simulink model "Modelo_nolineal_2GDL_2021"  (R2021b)
settings: Solver=VariableStepAuto  StartTime=0.0  StopTime=5  FixedStep=T  RelTol=1e-3
values from neighbouring files (symbols this model uses):
  g = 9.81    [initializationControl.m]
  Iyy = pod.mass.inertia(2,2)    [initializationControl.m]
  m = pod.mass.mass    [initializationControl.m]
  theta0 = 0    [initializationControl.m]
  x_lev = pod.geometry.x_LEV    [initializationControl.m]
  z_ini = z_0 + z_lev    [initializationControl.m]
  z_lev = pod.geometry.z_LEV    [initializationControl.m]
undefined symbols (not defined in the file or in its folder): k1, k2, k3, k4, p1, p2
settings Model: Creator=EDMAOR  LastModifiedBy=emate
settings SolverCC: AlgebraicLoopSolver=TrustRegion
settings DebuggingCC: SFMachineParentedDataDiag=warning
settings SFSimCC: CustomCodeUndefinedFunction=UseInterfaceOnly

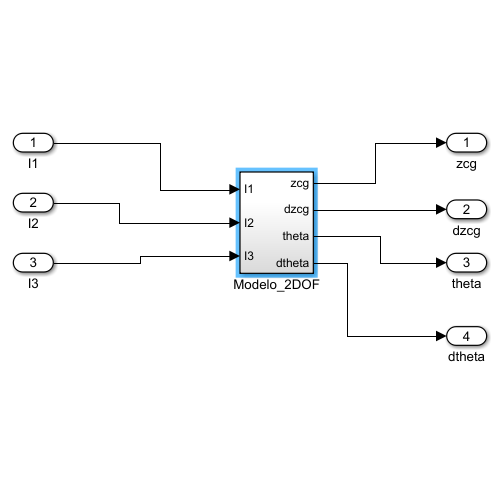
[thumbnail: Simulink's stored preview of the top-level diagram]
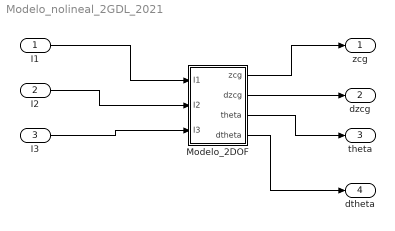
== system Modelo_nolineal_2GDL_2021 ==
  I1 : Inport
  I2 : Inport  Port=2
  I3 : Inport  Port=3
  Modelo_2DOF : Subsystem
  zcg : Outport  VectorParamsAs1DForOutWhenUnconnected=off
  dzcg : Outport  Port=2  VectorParamsAs1DForOutWhenUnconnected=off
  theta : Outport  Port=3  VectorParamsAs1DForOutWhenUnconnected=off
  dtheta : Outport  Port=4  VectorParamsAs1DForOutWhenUnconnected=off
  wires:
  Modelo_2DOF/1(zcg) -> zcg/1
  Modelo_2DOF/2(dzcg) -> dzcg/1
  I1/1 -> Modelo_2DOF/1(I1)
  I2/1 -> Modelo_2DOF/2(I2)
  I3/1 -> Modelo_2DOF/3(I3)
  Modelo_2DOF/3(theta) -> theta/1
  Modelo_2DOF/4(dtheta) -> dtheta/1

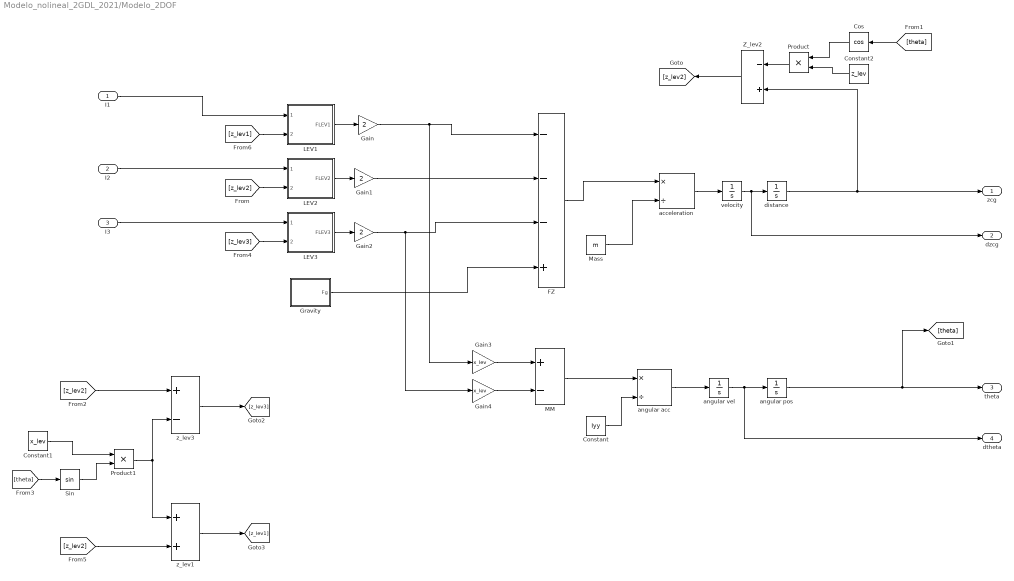
== system Modelo_nolineal_2GDL_2021/Modelo_2DOF ==
  I1 : Inport
  I2 : Inport  Port=2
  I3 : Inport  Port=3
  Constant : Constant  Value=Iyy
  Constant1 : Constant  Value=x_lev
  Constant2 : Constant  Value=z_lev
  Cos : Trigonometry  Operator=cos
  FZ : Sum  Inputs=---+
  Gain : Gain  Gain=2
  Gain1 : Gain  Gain=2
  Gain2 : Gain  Gain=2
  Gain3 : Gain  Gain=x_lev
  Gain4 : Gain  Gain=x_lev
  Gravity : Subsystem
  LEV1 : Subsystem
  LEV2 : Subsystem
  LEV3 : Subsystem
  MM : Sum  Inputs=+-
  Mass : Constant  Value=m
  Product : Product
  Product1 : Product
  Sin : Trigonometry
  Z_lev2 : Sum  Inputs=-+
  acceleration : Product  Inputs=*/
  angular acc : Product  Inputs=*/
  angular pos : Integrator  InitialCondition=theta0
  angular vel : Integrator
  distance : Integrator  InitialCondition=z_ini
  velocity : Integrator
  z_lev1 : Sum
  z_lev3 : Sum  Inputs=+-
  zcg : Outport  VectorParamsAs1DForOutWhenUnconnected=off
  dzcg : Outport  Port=2  VectorParamsAs1DForOutWhenUnconnected=off
  theta : Outport  Port=3  VectorParamsAs1DForOutWhenUnconnected=off
  dtheta : Outport  Port=4  VectorParamsAs1DForOutWhenUnconnected=off
  wires:
  acceleration/1 -> velocity/1
  velocity/1 -> dzcg/1, distance/1
  distance/1 -> Z_lev2/2, zcg/1
  I1/1 -> LEV1/1(current1)
  I2/1 -> LEV2/1(current2)
  I3/1 -> LEV3/1(current3)
  LEV1/1(FLEV1) -> Gain/1
  Gain/1 -> Gain3/1, FZ/1
  LEV2/1(FLEV2) -> Gain1/1
  Gain1/1 -> FZ/2
  LEV3/1(FLEV3) -> Gain2/1
  Gain2/1 -> Gain4/1, FZ/3
  Gravity/1(Fg) -> FZ/4
  FZ/1 -> acceleration/1
  Mass/1 -> acceleration/2
  Gain3/1 -> MM/1
  Gain4/1 -> MM/2
  MM/1 -> angular acc/1
  Constant/1 -> angular acc/2
  angular acc/1 -> angular vel/1
  angular vel/1 -> dtheta/1, angular pos/1
  angular pos/1 -> [theta], theta/1
  [z_lev2] -> LEV2/2(distance2)
  Cos/1 -> Product/1
  Constant2/1 -> Product/2
  Product/1 -> Z_lev2/1
  Z_lev2/1 -> [z_lev2]
  [theta] -> Cos/1
  [z_lev2] -> z_lev3/1
  [theta] -> Sin/1
  Sin/1 -> Product1/2
  Constant1/1 -> Product1/1
  Product1/1 -> z_lev3/2, z_lev1/1
  z_lev3/1 -> [z_lev3]
  [z_lev3] -> LEV3/2(distance3)
  [z_lev2] -> z_lev1/2
  z_lev1/1 -> [z_lev1]
  [z_lev1] -> LEV1/2(distance1)

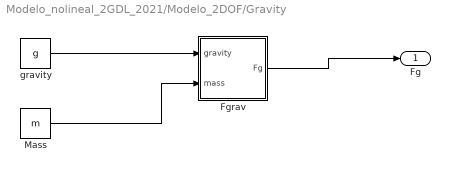
== system Modelo_nolineal_2GDL_2021/Modelo_2DOF/Gravity ==
  Fgrav : Subsystem
  Mass : Constant  Value=m
  gravity : Constant  Value=g
  Fg : Outport
  wires:
  Fgrav/1(Fg) -> Fg/1
  gravity/1 -> Fgrav/1(gravity)
  Mass/1 -> Fgrav/2(mass)

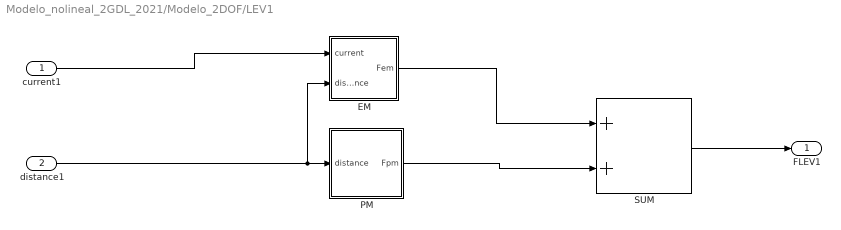
== system Modelo_nolineal_2GDL_2021/Modelo_2DOF/LEV1 ==
  current1 : Inport
  distance1 : Inport  Port=2
  EM : Subsystem
  PM : Subsystem
  SUM : Sum
  FLEV1 : Outport  VectorParamsAs1DForOutWhenUnconnected=off
  wires:
  PM/1(Fpm) -> SUM/2
  distance1/1 -> EM/2(distance), PM/1(distance)
  EM/1(Fem) -> SUM/1
  current1/1 -> EM/1(current)
  SUM/1 -> FLEV1/1

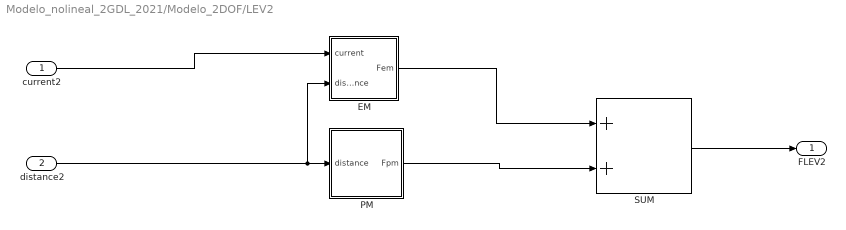
== system Modelo_nolineal_2GDL_2021/Modelo_2DOF/LEV2 ==
  current2 : Inport
  distance2 : Inport  Port=2
  EM : Subsystem
  PM : Subsystem
  SUM : Sum
  FLEV2 : Outport  VectorParamsAs1DForOutWhenUnconnected=off
  wires:
  SUM/1 -> FLEV2/1
  current2/1 -> EM/1(current)
  EM/1(Fem) -> SUM/1
  distance2/1 -> PM/1(distance), EM/2(distance)
  PM/1(Fpm) -> SUM/2

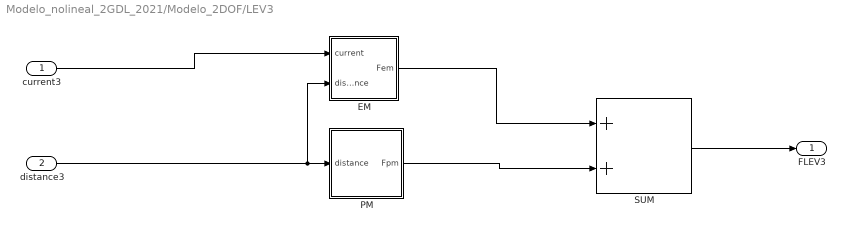
== system Modelo_nolineal_2GDL_2021/Modelo_2DOF/LEV3 ==
  current3 : Inport
  distance3 : Inport  Port=2
  EM : Subsystem
  PM : Subsystem
  SUM : Sum
  FLEV3 : Outport  VectorParamsAs1DForOutWhenUnconnected=off
  wires:
  PM/1(Fpm) -> SUM/2
  distance3/1 -> EM/2(distance), PM/1(distance)
  EM/1(Fem) -> SUM/1
  current3/1 -> EM/1(current)
  SUM/1 -> FLEV3/1

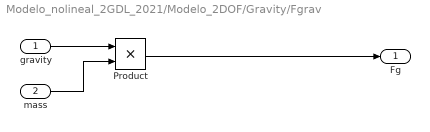
== system Modelo_nolineal_2GDL_2021/Modelo_2DOF/Gravity/Fgrav ==
  gravity : Inport
  mass : Inport  Port=2
  Product : Product
  Fg : Outport  VectorParamsAs1DForOutWhenUnconnected=off
  wires:
  Product/1 -> Fg/1
  gravity/1 -> Product/1
  mass/1 -> Product/2

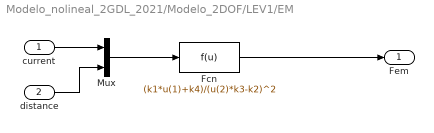
== system Modelo_nolineal_2GDL_2021/Modelo_2DOF/LEV1/EM ==
  current : Inport
  distance : Inport  Port=2
  Fcn : Fcn  Expr=(k1*u(1)+k4)/(u(2)*k3-k2)^2
  Mux : Mux  Inputs=2
  Fem : Outport  VectorParamsAs1DForOutWhenUnconnected=off
  wires:
  current/1 -> Mux/1
  distance/1 -> Mux/2
  Mux/1 -> Fcn/1
  Fcn/1 -> Fem/1

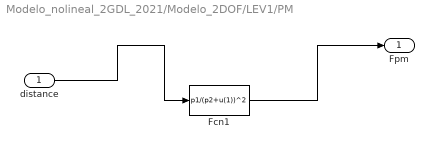
== system Modelo_nolineal_2GDL_2021/Modelo_2DOF/LEV1/PM ==
  distance : Inport
  Fcn1 : Fcn  Expr=p1/(p2+u(1))^2
  Fpm : Outport  VectorParamsAs1DForOutWhenUnconnected=off
  wires:
  distance/1 -> Fcn1/1
  Fcn1/1 -> Fpm/1

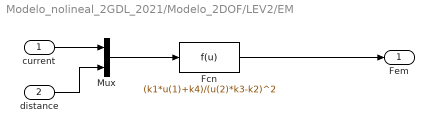
== system Modelo_nolineal_2GDL_2021/Modelo_2DOF/LEV2/EM ==
  current : Inport
  distance : Inport  Port=2
  Fcn : Fcn  Expr=(k1*u(1)+k4)/(u(2)*k3-k2)^2
  Mux : Mux  Inputs=2
  Fem : Outport  VectorParamsAs1DForOutWhenUnconnected=off
  wires:
  Fcn/1 -> Fem/1
  Mux/1 -> Fcn/1
  distance/1 -> Mux/2
  current/1 -> Mux/1

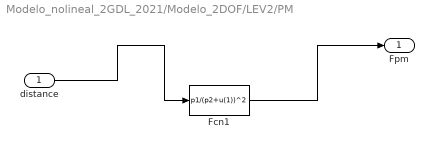
== system Modelo_nolineal_2GDL_2021/Modelo_2DOF/LEV2/PM ==
  distance : Inport
  Fcn1 : Fcn  Expr=p1/(p2+u(1))^2
  Fpm : Outport  VectorParamsAs1DForOutWhenUnconnected=off
  wires:
  Fcn1/1 -> Fpm/1
  distance/1 -> Fcn1/1

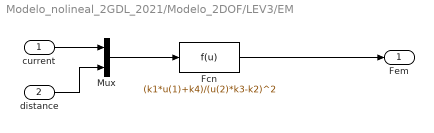
== system Modelo_nolineal_2GDL_2021/Modelo_2DOF/LEV3/EM ==
  current : Inport
  distance : Inport  Port=2
  Fcn : Fcn  Expr=(k1*u(1)+k4)/(u(2)*k3-k2)^2
  Mux : Mux  Inputs=2
  Fem : Outport  VectorParamsAs1DForOutWhenUnconnected=off
  wires:
  current/1 -> Mux/1
  distance/1 -> Mux/2
  Mux/1 -> Fcn/1
  Fcn/1 -> Fem/1

== system Modelo_nolineal_2GDL_2021/Modelo_2DOF/LEV3/PM ==
  distance : Inport
  Fcn1 : Fcn  Expr=p1/(p2+u(1))^2
  Fpm : Outport  VectorParamsAs1DForOutWhenUnconnected=off
  wires:
  distance/1 -> Fcn1/1
  Fcn1/1 -> Fpm/1
